simulink model "sat_Sim_V_in"  (R2024b)
settings: Solver=VariableStepAuto  StartTime=0.0  StopTime=20  RelTol=1e-3
values from neighbouring files (symbols this model uses):
  h = -600000    [main.m]
  phi_in = (0)*(pi/180)    (= 0)    [main.m]
  psi_in = (90)*(pi/180)    (= 1.57079632679)    [main.m]
  theta_in = (45)*(pi/180)    (= 0.785398163397)    [main.m]
undefined symbols (not defined in the file or in its folder): Earth, motor, sat, WGS84
libraries: slpidlib x3, aerolibfltsims x2, aerolibsim3d x2, aerolibtransform2 x1, aerolibanim x1, sim3dlib x1
settings Model: Creator=ben  LastModifiedBy=ben

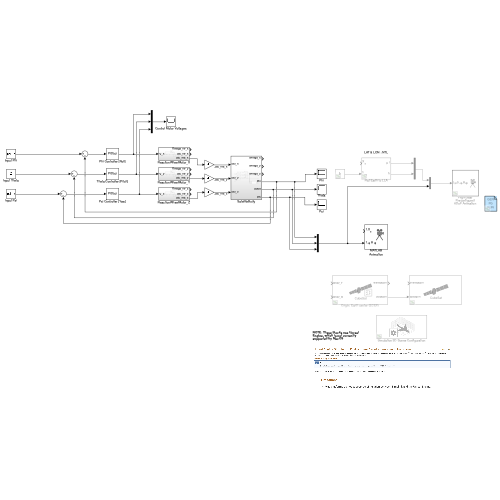
[thumbnail: Simulink's stored preview of the top-level diagram]
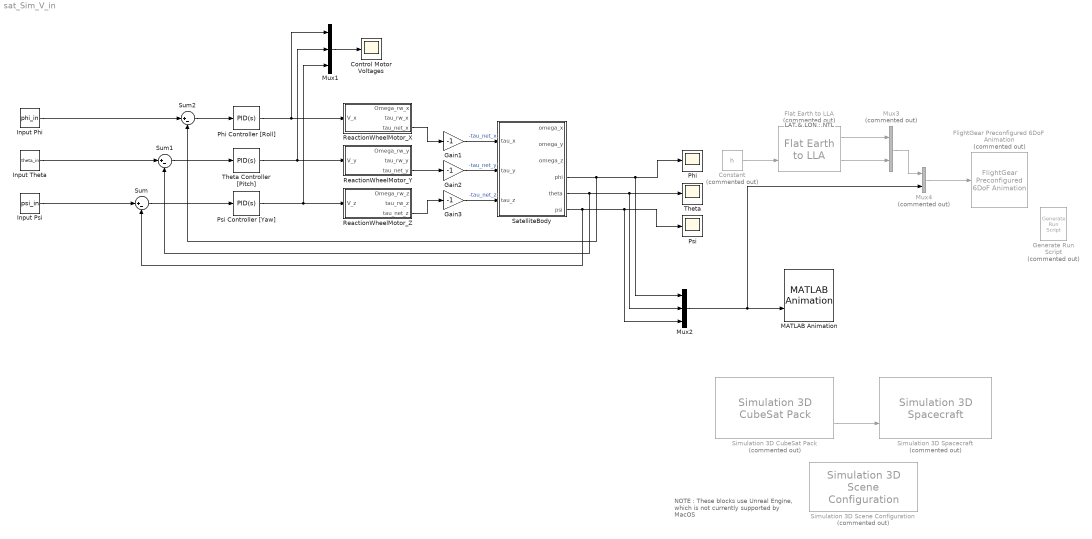
== system sat_Sim_V_in ==
  note: LAT & LON : NTL
  note: NOTE : These blocks use Unreal Engine, which is not currently supported by MacOS
  Constant : Constant  Commented=on  Value=h
  Control Motor Voltages : Scope
  Flat Earth to LLA : aerolibtransform2/Flat Earth to LLA  Commented=on  units=Metric (MKS)  ptype=Earth (WGS84)  F=1/298.257223563  R=6378137  refPosPort=off  LL0=[22 150]  psi=0
  FlightGear Preconfigured 6DoF Animation : aerolibfltsims/FlightGear Preconfigured 6DoF Animation  Commented=on  xFlightGearVersion=v2019.1  DestinationIpAddress=127.0.0.1  DestinationPort=5502  SampleTime=1/20  packetVersion=24
  Gain1 : Gain  Gain=-1
  Gain2 : Gain  Gain=-1
  Gain3 : Gain  Gain=-1
  Generate Run Script : aerolibfltsims/Generate Run Script  Commented=on  Architecture=Mac  dataFlow=Send  GeometryModelName=c172p  AirportId=YSSY  RunwayId=10L  InitialAltitude=7224  InitialHeading=113  OffsetDistance=4.72  OffsetAzimuth=0  InstallScenery=on  DisableShaders=on  OriginAddress=127.0.0.1  DestinationPort=5502  OriginPort=5505  LocalAddress=127.0.0.1  OutputFileName=runfg2.sh  FlightGearBaseDirectory=/Applications/FlightGear.app
  Input Phi : Constant  Value=phi_in  SampleTime=0.1
  Input Psi : Constant  Value=psi_in
  Input Theta : Constant  Value=theta_in
  MATLAB Animation : aerolibanim/MATLAB Animation  Tag=Matlab Animation 6 DOF  Vehicles=1  Geometries='pa24-250_orange.ac'  BoundingBoxCoordinates=[-50,50,-50,50,-50,50]  CameraOffset=[-150,0,0]  CameraViewAngle=5  SampleTime=0.01  FigurePosition=[761,102,744,779]
  Mux1 : Mux  Inputs=3
  Mux2 : Mux  Inputs=3
  Mux3 : Mux  Commented=on  Inputs=2
  Mux4 : Mux  Commented=on  Inputs=2
  Phi : Scope
  Phi Controller [Roll] : slpidlib/PID Controller  Controller=PID  Form=Parallel  TimeDomain=Continuous-time  UseExternalTs=off  SampleTime=-1  IntegratorMethod=Forward Euler  FilterMethod=Forward Euler  ControllerParametersSource=internal  P=-50.4825434106595  I=-1.23008759816909  UseKiTs=off  D=-412.023535687071  UseExternalDerivativeSource=off  N=0.379397383172155  UseFilter=on  TunerSelectOption=Transfer Function Based (PID Tuner App)  InitialConditionSource=internal  InitialConditionForIntegrator=0  InitialConditionForFilter=0  DifferentiatorICPrevScaledInput=0  ExternalReset=none  TrackingMode=off  Kt=1  LimitOutput=off  SatLimitsSource=internal  UpperSaturationLimit=inf  LowerSaturationLimit=-inf  LinearizeAsGain=on  AntiWindupMode=none  Kb=1  LimitIntegrator=off  UpperIntegratorSaturationLimit=inf  LowerIntegratorSaturationLimit=-inf  POutMin=[]  POutMax=[]  IOutMin=[]  IOutMax=[]  DOutMin=[]  DOutMax=[]  NOutMin=[]  NOutMax=[]  SumOutMin=[]  SumOutMax=[]  SaturationOutMin=[]  SaturationOutMax=[]  PParamMin=[]  PParamMax=[]  IParamMin=[]  IParamMax=[]  DParamMin=[]  DParamMax=[]  NParamMin=[]  NParamMax=[]  KbParamMin=[]  KbParamMax=[]  KtParamMin=[]  KtParamMax=[]  KbOutMin=[]  KbOutMax=[]  KtOutMin=[]  KtOutMax=[]  IntegratorOutMin=[]  IntegratorOutMax=[]  FilterOutMin=[]  FilterOutMax=[]  SumI1OutMin=[]  SumI1OutMax=[]  SumI2OutMin=[]  SumI2OutMax=[]  SumI3OutMin=[]  SumI3OutMax=[]  SumI4OutMin=[]  SumI4OutMax=[]  SumDOutMin=[]  SumDOutMax=[]  DifferentiatorOutMin=[]  DifferentiatorOutMax=[]  FilterDiffOutCoefMin=[]  FilterDiffOutCoefMax=[]  ReciprocalOutMin=[]  ReciprocalOutMax=[]  SumDenOutMin=[]  SumDenOutMax=[]  SumNumOutMin=[]  SumNumOutMax=[]  DivideOutMin=[]  DivideOutMax=[]  UdiffTsProdOutMin=[]  UdiffTsProdOutMax=[]  NTsProdOutMin=[]  NTsProdOutMax=[]  UintegralTsProdOutMin=[]  UintegralTsProdOutMax=[]  UngainTsProdOutMin=[]  UngainTsProdOutMax=[]  ClampingZeroOutDataTypeStr=Inherit: Inherit via back propagation  ClampingZeroOutMin=[]  ClampingZeroOutMax=[]  FilterDenConstantOutDataTypeStr=Inherit: Inherit via back propagation  FilterDenConstantOutMin=[]  FilterDenConstantOutMax=[]  PCopyOutDataTypeStr=Inherit: Inherit via back propagation  PCopyOutMin=[]  PCopyOutMax=[]  NCopyOutDataTypeStr=Inherit: Inherit via back propagation  NCopyOutMin=[]  NCopyOutMax=[]  IntegratorContinuousStateAttributes=''  IntegratorStateMustResolveToSignalObject=off  IntegratorRTWStateStorageClass=Auto  FilterContinuousStateAttributes=''  FilterStateMustResolveToSignalObject=off  FilterRTWStateStorageClass=Auto  ParallelPVariant=InternalParameters  IdealPVariant=Disabled  IVariant=InternalParameters  DVariant=InternalParameters  IntegratorVariant=Continuous  SatVariant=Disabled  AWVariant=Passthrough  PCopyVariant=Disabled  TRVariant=Disabled  FdbkBlocksVariant=Forward  IdealPFdbkVariant=Disabled  SatFdbkVariant=Disabled  DerivativeFilterVariant=ContFilter  NVariant=InternalParameters  NCopyVariant=Disabled  FilterICVariant=InternalICsFilter  IntegratorICVariant=InternalICs  ExternalResetVariant=Disabled  TRSumVariant=Passthrough  SumFdbkVariant=Disabled  SumVariant=Sum_PID  TsampFilterVariant=InternalTs  TsampNgainVariant=Passthrough  TsampIntegralVariant=Disabled_SignalSpec  ExternalSaturationOutDataTypeStr=Inherit: Same as second input  DerivativeSourceVariant=ErrorSignal  PreIntVariant=InternalPreInt
  Psi : Scope
  Psi Controller [Yaw] : slpidlib/PID Controller  Controller=PID  Form=Parallel  TimeDomain=Continuous-time  UseExternalTs=off  SampleTime=-1  IntegratorMethod=Forward Euler  FilterMethod=Forward Euler  ControllerParametersSource=internal  P=-763.325878025154  I=-72.3330718489805  UseKiTs=off  D=-1552.13165448844  UseExternalDerivativeSource=off  N=226.089930864036  UseFilter=on  TunerSelectOption=Transfer Function Based (PID Tuner App)  InitialConditionSource=internal  InitialConditionForIntegrator=0  InitialConditionForFilter=0  DifferentiatorICPrevScaledInput=0  ExternalReset=none  TrackingMode=off  Kt=1  LimitOutput=off  SatLimitsSource=internal  UpperSaturationLimit=inf  LowerSaturationLimit=-inf  LinearizeAsGain=on  AntiWindupMode=none  Kb=1  LimitIntegrator=off  UpperIntegratorSaturationLimit=inf  LowerIntegratorSaturationLimit=-inf  POutMin=[]  POutMax=[]  IOutMin=[]  IOutMax=[]  DOutMin=[]  DOutMax=[]  NOutMin=[]  NOutMax=[]  SumOutMin=[]  SumOutMax=[]  SaturationOutMin=[]  SaturationOutMax=[]  PParamMin=[]  PParamMax=[]  IParamMin=[]  IParamMax=[]  DParamMin=[]  DParamMax=[]  NParamMin=[]  NParamMax=[]  KbParamMin=[]  KbParamMax=[]  KtParamMin=[]  KtParamMax=[]  KbOutMin=[]  KbOutMax=[]  KtOutMin=[]  KtOutMax=[]  IntegratorOutMin=[]  IntegratorOutMax=[]  FilterOutMin=[]  FilterOutMax=[]  SumI1OutMin=[]  SumI1OutMax=[]  SumI2OutMin=[]  SumI2OutMax=[]  SumI3OutMin=[]  SumI3OutMax=[]  SumI4OutMin=[]  SumI4OutMax=[]  SumDOutMin=[]  SumDOutMax=[]  DifferentiatorOutMin=[]  DifferentiatorOutMax=[]  FilterDiffOutCoefMin=[]  FilterDiffOutCoefMax=[]  ReciprocalOutMin=[]  ReciprocalOutMax=[]  SumDenOutMin=[]  SumDenOutMax=[]  SumNumOutMin=[]  SumNumOutMax=[]  DivideOutMin=[]  DivideOutMax=[]  UdiffTsProdOutMin=[]  UdiffTsProdOutMax=[]  NTsProdOutMin=[]  NTsProdOutMax=[]  UintegralTsProdOutMin=[]  UintegralTsProdOutMax=[]  UngainTsProdOutMin=[]  UngainTsProdOutMax=[]  ClampingZeroOutDataTypeStr=Inherit: Inherit via back propagation  ClampingZeroOutMin=[]  ClampingZeroOutMax=[]  FilterDenConstantOutDataTypeStr=Inherit: Inherit via back propagation  FilterDenConstantOutMin=[]  FilterDenConstantOutMax=[]  PCopyOutDataTypeStr=Inherit: Inherit via back propagation  PCopyOutMin=[]  PCopyOutMax=[]  NCopyOutDataTypeStr=Inherit: Inherit via back propagation  NCopyOutMin=[]  NCopyOutMax=[]  IntegratorContinuousStateAttributes=''  IntegratorStateMustResolveToSignalObject=off  IntegratorRTWStateStorageClass=Auto  FilterContinuousStateAttributes=''  FilterStateMustResolveToSignalObject=off  FilterRTWStateStorageClass=Auto  ParallelPVariant=InternalParameters  IdealPVariant=Disabled  IVariant=InternalParameters  DVariant=InternalParameters  IntegratorVariant=Continuous  SatVariant=Disabled  AWVariant=Passthrough  PCopyVariant=Disabled  TRVariant=Disabled  FdbkBlocksVariant=Forward  IdealPFdbkVariant=Disabled  SatFdbkVariant=Disabled  DerivativeFilterVariant=ContFilter  NVariant=InternalParameters  NCopyVariant=Disabled  FilterICVariant=InternalICsFilter  IntegratorICVariant=InternalICs  ExternalResetVariant=Disabled  TRSumVariant=Passthrough  SumFdbkVariant=Disabled  SumVariant=Sum_PID  TsampFilterVariant=InternalTs  TsampNgainVariant=Passthrough  TsampIntegralVariant=Disabled_SignalSpec  ExternalSaturationOutDataTypeStr=Inherit: Same as second input  DerivativeSourceVariant=ErrorSignal  PreIntVariant=InternalPreInt
  ReactionWheelMotor_X : Subsystem
  ReactionWheelMotor_Y : Subsystem
  ReactionWheelMotor_Z : Subsystem
  SatelliteBody : Subsystem
  Simulation 3D CubeSat Pack : aerolibsim3d/Simulation 3D CubeSat Pack  Commented=on  Antenna1_T=off  Antenna1_R=off  Antenna2_T=off  Antenna2_R=off  Antenna3_T=off  Antenna3_R=off  Sensor_T=off  Sensor_R=off  SolarArray1_T=off  SolarArray1_R=off  SolarArray1_1_T=off  SolarArray1_1_R=off  SolarArray2_T=off  SolarArray2_R=off  SolarArray2_2_T=off  SolarArray2_2_R=off  Thruster_T=off  Thruster_R=off  GeoRadioButton=ECEF  AdjustForCesium=on  Heading0=90
      settings: AttributesFormatString=Origin: Earth center (ECEF)
  Simulation 3D Scene Configuration : sim3dlib/Simulation 3D Scene Configuration  Priority=0  Commented=on  ProjectFormat=Default Scenes  SceneDesc=Airport  ProjectName=B:\matlab\toolbox\shared\sim3d_projects\automotive_project_windows\UE\WindowsNoEditor\VehicleSimulation.exe  ScenePath=/Game/Maps/HwStrght  EnableOpenDRIVE=off  vehTagList={'Custom';'Scene Origin';'SimulinkVehicle1'}  vehTag=Scene Origin  FreeCameraInitialTranslation=[-6, 0, 2]  FreeCameraDefaultInitialTranslation=[-6, 0, 2]  FreeCameraInitialRotation=[0, -15, 0]  FreeCameraDefaultInitialRotation=[0, -15, 0]  OpVisEn=off  Ts=.02  EnableWindow=on  EnableRemoteAccess=off  EnableWeather=off  SunAzimuth=90  SunAltitude=40.0  EnableGeospatialSun=off  Latitude=0  Longitude=0  Date=2023-01-01  Time=10:30:00  GeoTimeZone=-5.0  SunDaylightSaving=off  wind=1  clouds=10  EnableVolumetricClouds=off  CloudCoverage=0  CloudAltitude=6  fog=0  rain=0  RaindropsEffect=off  SnowDensity=0  EnableGeospatial=off  UseTrueOrigin=off  OriginHeight=200  OriginLatitude=40.744652  OriginLongitude=-73.988864  MapStyle=Aerial  AdditionalAssetIDs=[]  UseAdvancedSunSky=off  SolarTime=11  TimeZone=-5  Day=21  Month=9  Year=2022  UseDaylightSavingTime=on  DSTStartDay=10  DSTStartMonth=3  DSTEndDay=3  DSTEndMonth=11  DSTSwitchHour=2  sensorTag=MainCamera1  sensorId=1  sensorName=MainCamera1  mountLoc=Origin  offsetFlag=off  tmountOffset=[0, 0, 0]  rmountOffset=[0, 0, 0]  HorizontalResolution=1280  VerticalResolution=720  HorizontalFOV=60  mountPoint=[0 0 0]  mountOrientation=[0 0 0]  aMode=0  ID=1  GeoTrigger=Inactive
      settings: LibrarySourceBlock=aerolibsim3d/Simulation 3D Scene Configuration
  Simulation 3D Spacecraft : aerolibsim3d/Simulation 3D Spacecraft  Priority=1  Commented=on  Mesh=CubeSat  MeshPath=/MathWorksAerospaceContent/Vehicles/Spacecraft/CubeSat/Mesh/SK_CubeSat.SK_CubeSat  MeshPathSmall=/MathWorksAerospaceContent/Vehicles/Spacecraft/SmallSat/Mesh/SK_SmallSat.SK_SmallSat  SpacecraftColor=Silver  ActorName=SimulinkVehicle1  Translation=zeros(10, 3)  Rotation=zeros(10, 3)  ScaleInputPort=Dialog  Scale=[1 1 1]  InitialScale=[1 1 1]  IsGHSensorEnabled=off  AreGHRaysVisible=off  IsOutputReshapeEnabled=on  GHRayLength=1524  GHBodyOffset=1  GHContactLocation1=[0 0 0]  GHContactLocation2=[0 0 0]  GHContactLocation3=[0 0 0]  GHContactLocation4=[0 0 0]  WoWSensorTolerance=0.05  SampleTime=-1  ActorType=SimulinkVehicle  ID=1  aMode=0  ActorTag=SimulinkVehicle1
  Sum : Sum  Inputs=|+-
  Sum1 : Sum  Inputs=|+-
  Sum2 : Sum  Inputs=|+-
  Theta : Scope
  Theta Controller [Pitch] : slpidlib/PID Controller  Controller=PID  Form=Parallel  TimeDomain=Continuous-time  UseExternalTs=off  SampleTime=-1  IntegratorMethod=Forward Euler  FilterMethod=Forward Euler  ControllerParametersSource=internal  P=-456.390816139374  I=-30.5631615457373  UseKiTs=off  D=-1701.86514883062  UseExternalDerivativeSource=off  N=163.363333487621  UseFilter=on  TunerSelectOption=Transfer Function Based (PID Tuner App)  InitialConditionSource=internal  InitialConditionForIntegrator=0  InitialConditionForFilter=0  DifferentiatorICPrevScaledInput=0  ExternalReset=none  TrackingMode=off  Kt=1  LimitOutput=off  SatLimitsSource=internal  UpperSaturationLimit=inf  LowerSaturationLimit=-inf  LinearizeAsGain=on  AntiWindupMode=none  Kb=1  LimitIntegrator=off  UpperIntegratorSaturationLimit=inf  LowerIntegratorSaturationLimit=-inf  POutMin=[]  POutMax=[]  IOutMin=[]  IOutMax=[]  DOutMin=[]  DOutMax=[]  NOutMin=[]  NOutMax=[]  SumOutMin=[]  SumOutMax=[]  SaturationOutMin=[]  SaturationOutMax=[]  PParamMin=[]  PParamMax=[]  IParamMin=[]  IParamMax=[]  DParamMin=[]  DParamMax=[]  NParamMin=[]  NParamMax=[]  KbParamMin=[]  KbParamMax=[]  KtParamMin=[]  KtParamMax=[]  KbOutMin=[]  KbOutMax=[]  KtOutMin=[]  KtOutMax=[]  IntegratorOutMin=[]  IntegratorOutMax=[]  FilterOutMin=[]  FilterOutMax=[]  SumI1OutMin=[]  SumI1OutMax=[]  SumI2OutMin=[]  SumI2OutMax=[]  SumI3OutMin=[]  SumI3OutMax=[]  SumI4OutMin=[]  SumI4OutMax=[]  SumDOutMin=[]  SumDOutMax=[]  DifferentiatorOutMin=[]  DifferentiatorOutMax=[]  FilterDiffOutCoefMin=[]  FilterDiffOutCoefMax=[]  ReciprocalOutMin=[]  ReciprocalOutMax=[]  SumDenOutMin=[]  SumDenOutMax=[]  SumNumOutMin=[]  SumNumOutMax=[]  DivideOutMin=[]  DivideOutMax=[]  UdiffTsProdOutMin=[]  UdiffTsProdOutMax=[]  NTsProdOutMin=[]  NTsProdOutMax=[]  UintegralTsProdOutMin=[]  UintegralTsProdOutMax=[]  UngainTsProdOutMin=[]  UngainTsProdOutMax=[]  ClampingZeroOutDataTypeStr=Inherit: Inherit via back propagation  ClampingZeroOutMin=[]  ClampingZeroOutMax=[]  FilterDenConstantOutDataTypeStr=Inherit: Inherit via back propagation  FilterDenConstantOutMin=[]  FilterDenConstantOutMax=[]  PCopyOutDataTypeStr=Inherit: Inherit via back propagation  PCopyOutMin=[]  PCopyOutMax=[]  NCopyOutDataTypeStr=Inherit: Inherit via back propagation  NCopyOutMin=[]  NCopyOutMax=[]  IntegratorContinuousStateAttributes=''  IntegratorStateMustResolveToSignalObject=off  IntegratorRTWStateStorageClass=Auto  FilterContinuousStateAttributes=''  FilterStateMustResolveToSignalObject=off  FilterRTWStateStorageClass=Auto  ParallelPVariant=InternalParameters  IdealPVariant=Disabled  IVariant=InternalParameters  DVariant=InternalParameters  IntegratorVariant=Continuous  SatVariant=Disabled  AWVariant=Passthrough  PCopyVariant=Disabled  TRVariant=Disabled  FdbkBlocksVariant=Forward  IdealPFdbkVariant=Disabled  SatFdbkVariant=Disabled  DerivativeFilterVariant=ContFilter  NVariant=InternalParameters  NCopyVariant=Disabled  FilterICVariant=InternalICsFilter  IntegratorICVariant=InternalICs  ExternalResetVariant=Disabled  TRSumVariant=Passthrough  SumFdbkVariant=Disabled  SumVariant=Sum_PID  TsampFilterVariant=InternalTs  TsampNgainVariant=Passthrough  TsampIntegralVariant=Disabled_SignalSpec  ExternalSaturationOutDataTypeStr=Inherit: Same as second input  DerivativeSourceVariant=ErrorSignal  PreIntVariant=InternalPreInt
  wires:
  Gain2/1 -> SatelliteBody/2(tau_y)  "-tau_net_y"
  Gain3/1 -> SatelliteBody/3(tau_z)  "-tau_net_z"
  ReactionWheelMotor_Y/3(tau_net_y) -> Gain2/1
  ReactionWheelMotor_Z/3(tau_net_z) -> Gain3/1
  ReactionWheelMotor_X/3(tau_net_x) -> Gain1/1
  Gain1/1 -> SatelliteBody/1(tau_x)  "-tau_net_x"
  Phi Controller [Roll]/1 -> Mux1/1, ReactionWheelMotor_X/1(V_x)
  Psi Controller [Yaw]/1 -> Mux1/3, ReactionWheelMotor_Z/1(V_z)
  Theta Controller [Pitch]/1 -> Mux1/2, ReactionWheelMotor_Y/1(V_y)
  Sum2/1 -> Phi Controller [Roll]/1
  Sum1/1 -> Theta Controller [Pitch]/1
  Sum/1 -> Psi Controller [Yaw]/1
  SatelliteBody/4(phi) -> Sum2/2, Mux2/1, Phi/1
  SatelliteBody/5(theta) -> Mux2/2, Theta/1, Sum1/2
  SatelliteBody/6(psi) -> Sum/2, Mux2/3, Psi/1
  Input Phi/1 -> Sum2/1
  Input Psi/1 -> Sum/1
  Input Theta/1 -> Sum1/1
  Mux1/1 -> Control Motor Voltages/1
  Simulation 3D CubeSat Pack/2 -> Simulation 3D Spacecraft/2
  Mux4/1 -> FlightGear Preconfigured 6DoF Animation/1
  Mux3/1 -> Mux4/1
  Mux2/1 -> MATLAB Animation/2, Mux4/2
  Flat Earth to LLA/2 -> Mux3/2
  Constant/1 -> Flat Earth to LLA/2
  Flat Earth to LLA/1 -> Mux3/1

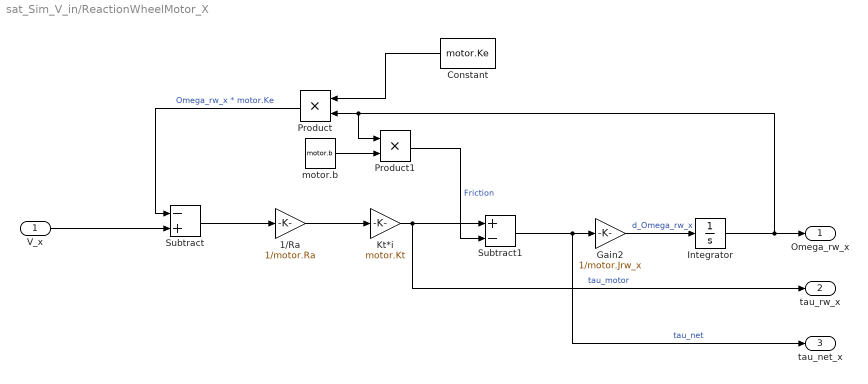
== system sat_Sim_V_in/ReactionWheelMotor_X ==
  V_x : Inport
  1/Ra : Gain  Gain=1/motor.Ra
  Constant : Constant  Value=motor.Ke
  Gain2 : Gain  Gain=1/motor.Jrw_x
  Integrator : Integrator
  Kt*i : Gain  Gain=motor.Kt
  Product : Product
  Product1 : Product
  Subtract : Sum  Inputs=-+
  Subtract1 : Sum  Inputs=+-
  motor.b : Constant  Value=motor.b  VectorParams1D=off
  Omega_rw_x : Outport
  tau_rw_x : Outport  Port=2
  tau_net_x : Outport  Port=3
  wires:
  Subtract1/1 -> tau_net_x/1, Gain2/1  "tau_net"
  Constant/1 -> Product/1
  V_x/1 -> Subtract/2
  Product/1 -> Subtract/1  "Omega_rw_x * motor.Ke"
  1/Ra/1 -> Kt*i/1
  Kt*i/1 -> Subtract1/1, tau_rw_x/1  "tau_motor"
  motor.b/1 -> Product1/2
  Product1/1 -> Subtract1/2  "Friction"
  Gain2/1 -> Integrator/1  "d_Omega_rw_x"
  Integrator/1 -> Product1/1, Product/2, Omega_rw_x/1
  Subtract/1 -> 1/Ra/1

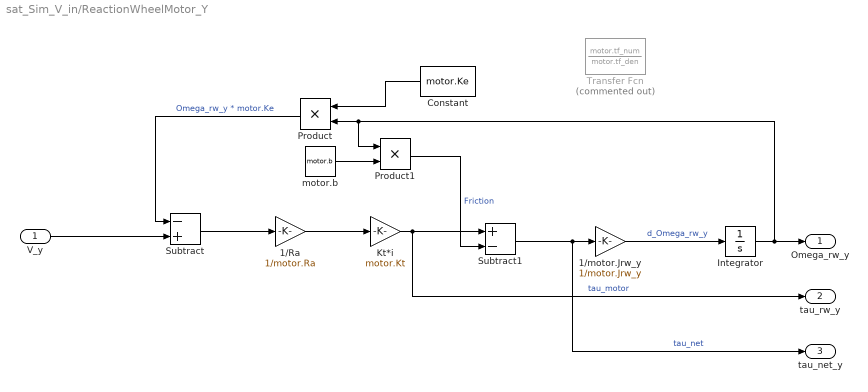
== system sat_Sim_V_in/ReactionWheelMotor_Y ==
  V_y : Inport
  1/Ra : Gain  Gain=1/motor.Ra
  1/motor.Jrw_y : Gain  Gain=1/motor.Jrw_y
  Constant : Constant  Value=motor.Ke
  Integrator : Integrator
  Kt*i : Gain  Gain=motor.Kt
  Product : Product
  Product1 : Product
  Subtract : Sum  Inputs=-+
  Subtract1 : Sum  Inputs=+-
  Transfer Fcn : TransferFcn  Commented=on  Numerator=motor.tf_num  Denominator=motor.tf_den
  motor.b : Constant  Value=motor.b  VectorParams1D=off
  Omega_rw_y : Outport
  tau_rw_y : Outport  Port=2
  tau_net_y : Outport  Port=3
  wires:
  Subtract1/1 -> tau_net_y/1, 1/motor.Jrw_y/1  "tau_net"
  Constant/1 -> Product/1
  V_y/1 -> Subtract/2
  Product/1 -> Subtract/1  "Omega_rw_y * motor.Ke"
  1/Ra/1 -> Kt*i/1
  Kt*i/1 -> Subtract1/1, tau_rw_y/1  "tau_motor"
  motor.b/1 -> Product1/2
  Product1/1 -> Subtract1/2  "Friction"
  1/motor.Jrw_y/1 -> Integrator/1  "d_Omega_rw_y"
  Integrator/1 -> Product1/1, Product/2, Omega_rw_y/1
  Subtract/1 -> 1/Ra/1

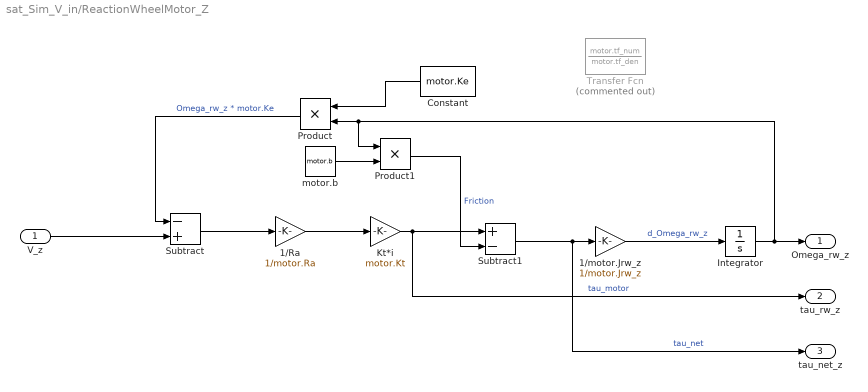
== system sat_Sim_V_in/ReactionWheelMotor_Z ==
  V_z : Inport
  1/Ra : Gain  Gain=1/motor.Ra
  1/motor.Jrw_z : Gain  Gain=1/motor.Jrw_z
  Constant : Constant  Value=motor.Ke
  Integrator : Integrator
  Kt*i : Gain  Gain=motor.Kt
  Product : Product
  Product1 : Product
  Subtract : Sum  Inputs=-+
  Subtract1 : Sum  Inputs=+-
  Transfer Fcn : TransferFcn  Commented=on  Numerator=motor.tf_num  Denominator=motor.tf_den
  motor.b : Constant  Value=motor.b  VectorParams1D=off
  Omega_rw_z : Outport
  tau_rw_z : Outport  Port=2
  tau_net_z : Outport  Port=3
  wires:
  Subtract1/1 -> tau_net_z/1, 1/motor.Jrw_z/1  "tau_net"
  Constant/1 -> Product/1
  V_z/1 -> Subtract/2
  Product/1 -> Subtract/1  "Omega_rw_z * motor.Ke"
  1/Ra/1 -> Kt*i/1
  Kt*i/1 -> Subtract1/1, tau_rw_z/1  "tau_motor"
  motor.b/1 -> Product1/2
  Product1/1 -> Subtract1/2  "Friction"
  1/motor.Jrw_z/1 -> Integrator/1  "d_Omega_rw_z"
  Integrator/1 -> Product1/1, Product/2, Omega_rw_z/1
  Subtract/1 -> 1/Ra/1

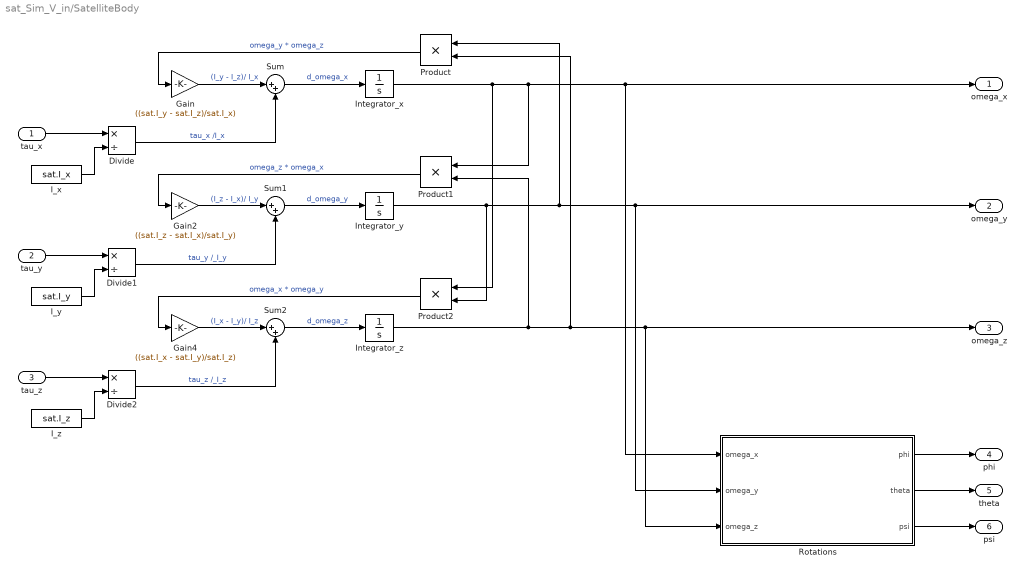
== system sat_Sim_V_in/SatelliteBody ==
  tau_x : Inport
  tau_y : Inport  Port=2
  tau_z : Inport  Port=3
  Divide : Product  Inputs=*/
  Divide1 : Product  Inputs=*/
  Divide2 : Product  Inputs=*/
  Gain : Gain  Gain=((sat.I_y - sat.I_z)/sat.I_x)
  Gain2 : Gain  Gain=((sat.I_z - sat.I_x)/sat.I_y)
  Gain4 : Gain  Gain=((sat.I_x - sat.I_y)/sat.I_z)
  I_x : Constant  Value=sat.I_x
  I_y : Constant  Value=sat.I_y
  I_z : Constant  Value=sat.I_z
  Integrator_x : Integrator
  Integrator_y : Integrator
  Integrator_z : Integrator
  Product : Product
  Product1 : Product
  Product2 : Product
  Rotations : Subsystem
  Sum : Sum  Inputs=|++
  Sum1 : Sum  Inputs=|++
  Sum2 : Sum  Inputs=|++
  omega_x : Outport
  omega_y : Outport  Port=2
  omega_z : Outport  Port=3
  phi : Outport  Port=4
  theta : Outport  Port=5
  psi : Outport  Port=6
  wires:
  Sum/1 -> Integrator_x/1  "d_omega_x"
  Integrator_x/1 -> Rotations/1(omega_x), omega_x/1, Product1/1, Product2/1
  Gain/1 -> Sum/1  "(I_y - I_z)/ I_x"
  Divide/1 -> Sum/2  "tau_x /I_x"
  Product/1 -> Gain/1  "omega_y * omega_z"
  Divide1/1 -> Sum1/2  "tau_y /_I_y"
  Integrator_y/1 -> Product2/2, Product/1, Rotations/2(omega_y), omega_y/1
  Gain2/1 -> Sum1/1  "(I_z - I_x)/ I_y"
  Sum1/1 -> Integrator_y/1  "d_omega_y"
  Product1/1 -> Gain2/1  "omega_z * omega_x"
  Divide2/1 -> Sum2/2  "tau_z /_I_z"
  Integrator_z/1 -> Product/2, Rotations/3(omega_z), omega_z/1, Product1/2
  Gain4/1 -> Sum2/1  "(I_x - I_y)/ I_z"
  Sum2/1 -> Integrator_z/1  "d_omega_z"
  Product2/1 -> Gain4/1  "omega_x * omega_y"
  Rotations/1(phi) -> phi/1
  Rotations/2(theta) -> theta/1
  Rotations/3(psi) -> psi/1
  tau_x/1 -> Divide/1
  I_x/1 -> Divide/2
  tau_y/1 -> Divide1/1
  I_y/1 -> Divide1/2
  tau_z/1 -> Divide2/1
  I_z/1 -> Divide2/2

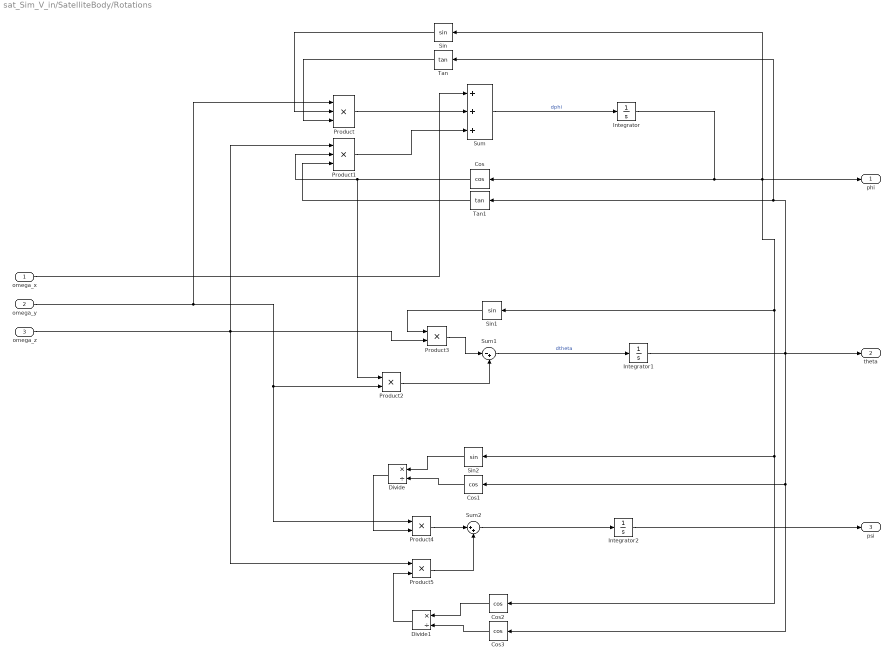
== system sat_Sim_V_in/SatelliteBody/Rotations ==
  omega_x : Inport
  omega_y : Inport  Port=2
  omega_z : Inport  Port=3
  Cos{,1..3} (4 alike) : Trigonometry  Operator=cos
  Divide : Product  Inputs=*/
  Divide1 : Product  Inputs=*/
  Integrator : Integrator
  Integrator1 : Integrator
  Integrator2 : Integrator
  Product : Product  Inputs=3
  Product1 : Product  Inputs=3
  Product{2..5} (4 alike) : Product
  Sin : Trigonometry
  Sin1 : Trigonometry
  Sin2 : Trigonometry
  Sum : Sum  Inputs=+++
  Sum1 : Sum  Inputs=|-+
  Sum2 : Sum  Inputs=|++
  Tan : Trigonometry  Operator=tan
  Tan1 : Trigonometry  Operator=tan
  phi : Outport
  theta : Outport  Port=2
  psi : Outport  Port=3
  wires:
  Integrator/1 -> Sin2/1, Cos2/1, Sin1/1, Sin/1, phi/1, Cos/1
  Integrator1/1 -> Cos1/1, Cos3/1, Tan1/1, Tan/1, theta/1
  Integrator2/1 -> psi/1
  Sum/1 -> Integrator/1  "dphi"
  Sum1/1 -> Integrator1/1  "dtheta"
  Sum2/1 -> Integrator2/1
  omega_x/1 -> Sum/1
  omega_y/1 -> Product/1, Product4/1, Product2/2
  Sin/1 -> Product/2
  Tan/1 -> Product/3
  Product/1 -> Sum/2
  Product1/1 -> Sum/3
  omega_z/1 -> Product5/1, Product3/2, Product1/1
  Cos/1 -> Product1/2, Product2/1
  Tan1/1 -> Product1/3
  Product2/1 -> Sum1/2
  Product3/1 -> Sum1/1
  Sin1/1 -> Product3/1
  Product4/1 -> Sum2/1
  Product5/1 -> Sum2/2
  Sin2/1 -> Divide/1
  Cos1/1 -> Divide/2
  Divide/1 -> Product4/2
  Divide1/1 -> Product5/2
  Cos2/1 -> Divide1/1
  Cos3/1 -> Divide1/2
